simulink model "MLIB_VAdd_BAM"  (Simulink 9.3)
settings: Solver=VariableStepAuto  StartTime=0.0  StopTime=10.0  RelTol=1e-3
settings Model: Creator=nxf41029  LastModifiedBy=nxf41029
settings DataIOCC: SaveFormat=Dataset  SignalLoggingSaveFormat=Dataset  ReturnWorkspaceOutputs=on
settings OptimizationCC: LifeSpan=auto
settings DebuggingCC: UnderspecifiedInitializationDetection=Simplified  MergeDetectMultiDrivingBlocksExec=error  FcnCallInpInsideContextMsg=error  SFUnexpectedBacktrackingDiag=error  SFNoUnconditionalDefaultTransitionDiag=error  SFExecutionAtInitializationDiag=warning  ArithmeticOperatorsInVariantConditions=error
settings HardwareCC: ProdBitPerPointer=64  ProdBitPerSizeT=64  ProdBitPerPtrDiffT=64  ProdLargestAtomicFloat=Float  ProdIntDivRoundTo=Zero  ProdEndianess=LittleEndian  ProdWordSize=64  ProdHWDeviceType=Intel->x86-64 (Windows64)
settings ModelReferenceCC: PropagateSignalLabelsOutOfModel=on
settings SFSimCC: SimUseLocalCustomCode=on
settings RTWCC: RTWUseLocalCustomCode=on
settings CodeAppCC: StateflowObjectComments=off
settings GRTTargetCC: TargetLangStandard=C99 (ISO)  CombineOutputUpdateFcns=on  GRTInterface=off
settings ConfigComp: CovMetricSettings=dwe  CovHtmlReporting=off  CovSaveCumulativeToWorkspaceVar=off  CovSaveSingleToWorkspaceVar=off  CovExternalEMLEnable=on

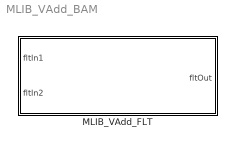
== system MLIB_VAdd_BAM ==
  MLIB_VAdd_FLT : Subsystem  TreatAsAtomicUnit=on  mask(MLIB_VAdd_FLT){}
      mask help: Vector addition in single precision floating-point implementation.
      mask init:
      | if ~evalin('base','exist(''tS8'',''var'')')
      |   if (2 ~= exist('SWLIBS_Typedefs.mat','file'))
      |       error('File SWLIBS_Typedefs.mat is not on the Matlab path. Please add the AMMCLIB "bam" folder in the Matlab Search Path.');
      |   else
      |       evalin('base', 'load(''SWLIBS_Typedefs.mat'')');
      |   end
      | end
      settings: RTWSystemCode=Inline
      mask Display: pos = get_param(gcb, 'Position');width = pos(3) - pos(1); height = pos(4) - pos(2);tX=width/2;tY=height - 8;color('black');text(tX,tY, 'MLIB_VAdd_FLT', 'horizontalAlignment', 'center');

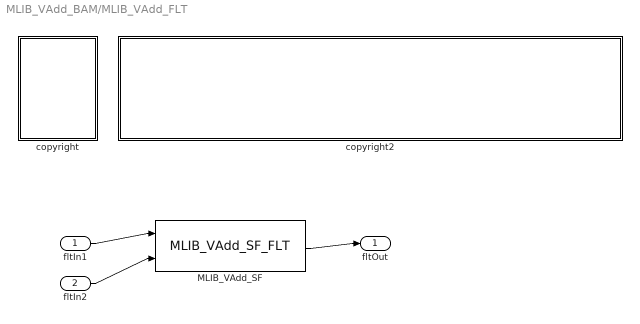
== system MLIB_VAdd_BAM/MLIB_VAdd_FLT ==
  fltIn1 : Inport  OutDataTypeStr=Bus: SWLIBS_2Syst_FLT  BusOutputAsStruct=on
  fltIn2 : Inport  Port=2  OutDataTypeStr=Bus: SWLIBS_2Syst_FLT  BusOutputAsStruct=on
  MLIB_VAdd_SF : S-Function  FunctionName=MLIB_VAdd_SF_FLT  SFunctionDeploymentMode=off  EnableBusSupport=off
  copyright : Subsystem
      mask Display: text(10,90,'FILE:');text(10,75,'DESRIPTION:');text(10,60,'COPYRIGHT:');text(10,45,'VERSION:');text(10,30,'DATE:')
  copyright2 : Subsystem
      mask Display: text(10,90,'MLIB_VAdd_BAM_FLT.mdl');text(10,75,'Vector addition.');text(10,60,'NXP 2020');text(10,45,'1.0');text(10,30,'28-May-2020');
  fltOut : Outport
  wires:
  fltIn1/1 -> MLIB_VAdd_SF/1
  fltIn2/1 -> MLIB_VAdd_SF/2
  MLIB_VAdd_SF/1 -> fltOut/1

== system MLIB_VAdd_BAM/MLIB_VAdd_FLT/copyright ==

== system MLIB_VAdd_BAM/MLIB_VAdd_FLT/copyright2 ==
